simulink model "Elevador"  (R2021a)
settings: Solver=VariableStepAuto  StartTime=0.0  StopTime=0.1  RelTol=1e-3
libraries: spsCurrentMeasurementLib x4, spsSeriesRLCBranchLib x3, spsVoltageMeasurementLib x2, spsDCVoltageSourceLib x1, spsDiodeLib x1, spsIdealSwitchLib x1, spspowerguiLib x1
settings Model: Creator=steve  LastModifiedBy=steve
settings SolverCC: AlgebraicLoopSolver=TrustRegion
settings DebuggingCC: SFMachineParentedDataDiag=warning

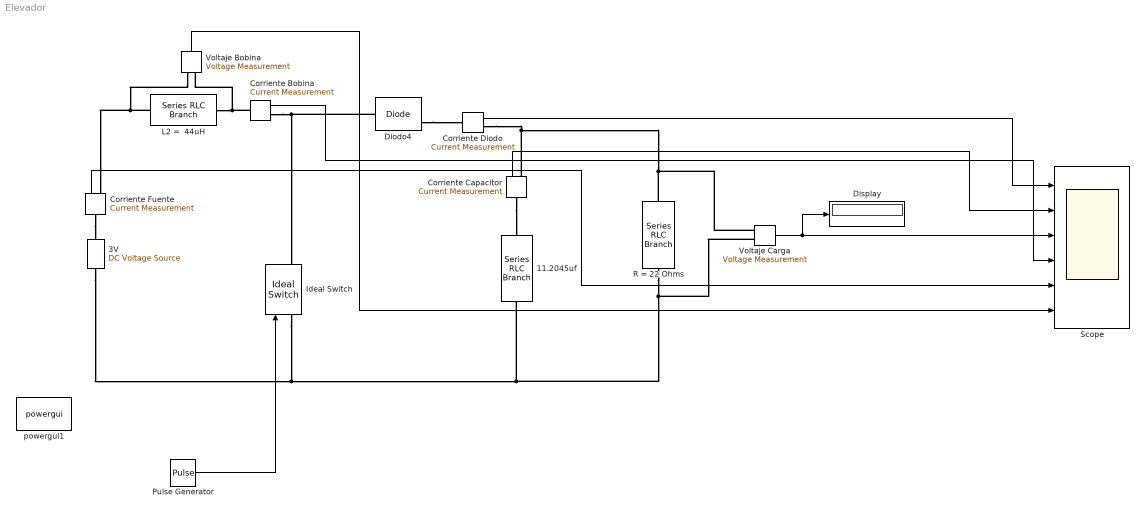
== system Elevador ==
  "11.2045uf " : spsSeriesRLCBranchLib/Series RLC Branch  LConnTagsString=__new0  RConnTagsString=__new0  BranchType=C  Resistance=100  Inductance=10  SetiL0=off  InitialCurrent=0  Capacitance=11.2045-6  Setx0=off  InitialVoltage=0  Measurements=None
  3V : spsDCVoltageSourceLib/DC Voltage Source  Amplitude=7  Measurements=None
  Corriente Bobina : spsCurrentMeasurementLib/Current Measurement  PhasorSimulation=off  OutputType=Complex  PSBequivalent=0
  Corriente Capacitor : spsCurrentMeasurementLib/Current Measurement  PhasorSimulation=off  OutputType=Complex  PSBequivalent=0
  Corriente Diodo : spsCurrentMeasurementLib/Current Measurement  PhasorSimulation=off  OutputType=Complex  PSBequivalent=0
  Corriente Fuente : spsCurrentMeasurementLib/Current Measurement  PhasorSimulation=off  OutputType=Complex  PSBequivalent=0
  Diodo4 : spsDiodeLib/Diode  Ron=0.001  Lon=0  Vf=.7  IC=0  UseSnubber=off  Rs=0  Cs=0  Measurements=on
  Display : Display
  Ideal Switch : spsIdealSwitchLib/Ideal Switch  Ron=0.001  Lon=0  IC=0  Rs=1e5  Cs=inf  Measurements=on
  L2 =  44uH : spsSeriesRLCBranchLib/Series RLC Branch  LConnTagsString=__new0  RConnTagsString=__new0  BranchType=L  Resistance=220  Inductance=44e-6  SetiL0=off  InitialCurrent=0  Capacitance=1e-6  Setx0=off  InitialVoltage=0  Measurements=None
  Pulse Generator : DiscretePulseGenerator  PulseType=Time based  Period=1/(20e3)  PulseWidth=20
  R = 22 Ohms : spsSeriesRLCBranchLib/Series RLC Branch  LConnTagsString=__new0  RConnTagsString=__new0  BranchType=R  Resistance=22  Inductance=1e-3  SetiL0=off  InitialCurrent=0  Capacitance=1e-6  Setx0=off  InitialVoltage=0  Measurements=None
  Scope : Scope  NumInputPorts=6
  Voltaje Bobina : spsVoltageMeasurementLib/Voltage Measurement  PhasorSimulation=off  OutputType=Complex  PSBequivalent=0
  Voltaje Carga : spsVoltageMeasurementLib/Voltage Measurement  PhasorSimulation=off  OutputType=Complex  PSBequivalent=0
  powergui1 : spspowerguiLib/powergui  Priority=1  SimulationMode=Continuous  SampleTime=50e-6  frequency=60  Iterations=50  frequencyindice=0  Pbase=100e6  ErrMax=1e-4  UnitsV=kV  UnitsW=MW  buscounter=0  FunctionMessages=off  echomessages=off  EnableUseOfTLC=off  CurrentSourceSwitches=off  DisableSnubberDevices=off  DisableRonSwitches=off  DisableVfSwitches=off  DisplayEquations=off  AutomaticDiscreteSolvers=off  SolverType=Tustin/Backward Euler (TBE)  Interpol=off  ExternalGateDelay=off  methode=off  Ts=100  x0status=blocks  SPID=on  SwTol=0  HookPort=off  NonlinearTolerance=1e-4  nMaxIteration=100  ContinueOnMaxIteration=off  RestoreLinks=warning  ResistiveCurrentMeasurement=off  Frange=[0:2:500]  Ylog=off  Xlog=on  ShowGrid=off  save=off  variable=ZData  structure=0  ZoomFFT=off  StartTime=0.0  cycles=1  DisplayStyle=1  fundamental=60  FreqAxis=off  MaxFrequency=1000  frequencyindicesteady=1  RmsSteady=1  display=off
  wires:
  Pulse Generator/1 -> Ideal Switch/1
  Voltaje Carga/1 -> Scope/3, Display/1
  Corriente Diodo/1 -> Scope/1
  Corriente Capacitor/1 -> Scope/2
  Corriente Fuente/1 -> Scope/5
  Voltaje Bobina/1 -> Scope/6
  Corriente Bobina/1 -> Scope/4
  connections:
  R = 22 Ohms/LConn1 -- Corriente Capacitor/RConn1 -- Corriente Diodo/RConn1 -- Voltaje Carga/LConn1
  L2 =  44uH/RConn1 -- Corriente Bobina/LConn1 -- Voltaje Bobina/LConn2
  R = 22 Ohms/RConn1 -- Voltaje Carga/LConn2 -- 3V/LConn1 -- Ideal Switch/LConn1 -- "11.2045uf "/RConn1
  Corriente Capacitor/LConn1 -- "11.2045uf "/LConn1
  Diodo4/RConn1 -- Corriente Diodo/LConn1
  Corriente Fuente/LConn1 -- 3V/RConn1
  L2 =  44uH/LConn1 -- Corriente Fuente/RConn1 -- Voltaje Bobina/LConn1
  Diodo4/LConn1 -- Ideal Switch/RConn1 -- Corriente Bobina/RConn1
